simulink model "Lab40DEGREE"  (R2020a)
settings: Solver=VariableStepAuto  StartTime=0.0  StopTime=0.1  RelTol=1e-3
libraries: powerlib x17
settings Model: Creator=Ahmad Raza  LastModifiedBy=Dell

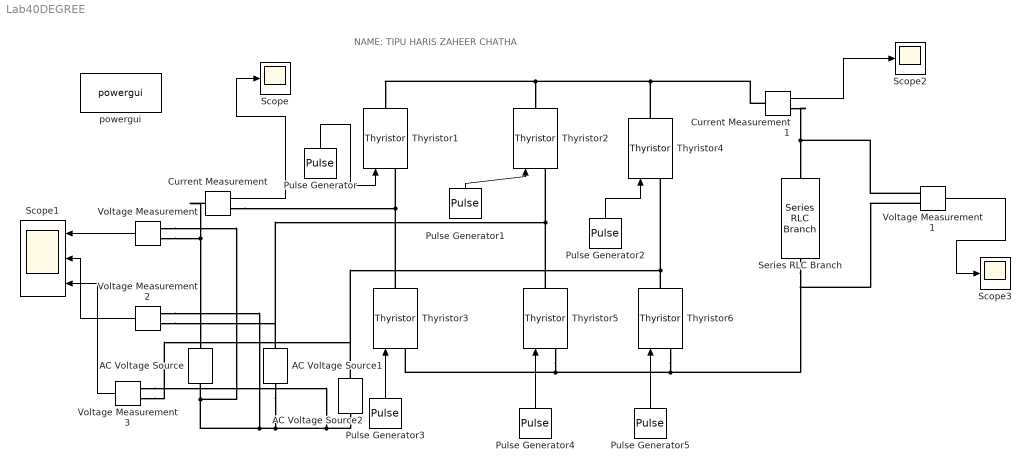
== system Lab40DEGREE ==
  note: NAME: TIPU HARIS ZAHEER CHATHA
  AC Voltage Source : powerlib/Electrical Sources/AC Voltage Source  Amplitude=100  Phase=0  Frequency=50  SampleTime=0  Measurements=None  BusType=swing  Pref=10e3  Qref=0  Qmin=-inf  Qmax=+inf
  AC Voltage Source1 : powerlib/Electrical Sources/AC Voltage Source  Amplitude=100  Phase=120  Frequency=50  SampleTime=0  Measurements=None  BusType=swing  Pref=10e3  Qref=0  Qmin=-inf  Qmax=+inf
  AC Voltage Source2 : powerlib/Electrical Sources/AC Voltage Source  Amplitude=100  Phase=240  Frequency=50  SampleTime=0  Measurements=None  BusType=swing  Pref=10e3  Qref=0  Qmin=-inf  Qmax=+inf
  Current Measurement : powerlib/Measurements/Current Measurement  PhasorSimulation=off  OutputType=Complex  PSBequivalent=0
  Current Measurement1 : powerlib/Measurements/Current Measurement  PhasorSimulation=off  OutputType=Complex  PSBequivalent=0
  Pulse Generator : DiscretePulseGenerator  PulseType=Time based  Amplitude=10  Period=0.02  PulseWidth=33.33  PhaseDelay=0/(360*50)
  Pulse Generator1 : DiscretePulseGenerator  PulseType=Time based  Amplitude=10  Period=0.02  PulseWidth=33.33  PhaseDelay=120/(360*50)
  Pulse Generator2 : DiscretePulseGenerator  PulseType=Time based  Amplitude=10  Period=0.02  PulseWidth=33.33  PhaseDelay=240/(360*50)
  Pulse Generator3 : DiscretePulseGenerator  PulseType=Time based  Amplitude=10  Period=0.02  PulseWidth=33.33  PhaseDelay=300/(360*50)
  Pulse Generator4 : DiscretePulseGenerator  PulseType=Time based  Amplitude=10  Period=0.02  PulseWidth=33.33  PhaseDelay=60/(360*50)
  Pulse Generator5 : DiscretePulseGenerator  PulseType=Time based  Amplitude=10  Period=0.02  PulseWidth=33.33  PhaseDelay=180/(360*50)
  Scope : Scope
  Scope1 : Scope  NumInputPorts=3
  Scope2 : Scope
  Scope3 : Scope
  Series RLC Branch : powerlib/Elements/Series RLC Branch  LConnTagsString=__new0  RConnTagsString=__new0  BranchType=R  Resistance=1  Inductance=1e-3  SetiL0=off  InitialCurrent=0  Capacitance=1e-6  Setx0=off  InitialVoltage=0  Measurements=None
  Thyristor{1..6} (6 alike) : powerlib/Power Electronics/Thyristor  Ron=0.001  Lon=0  Vf=0.8  IC=0  Rs=500  Cs=250e-9  Measurements=off
  Voltage Measurement{,1..3} (4 alike) : powerlib/Measurements/Voltage Measurement  PhasorSimulation=off  OutputType=Complex  PSBequivalent=0
  powergui : powerlib/powergui  Priority=1  SimulationMode=Continuous  SampleTime=50e-6  frequency=60  Iterations=50  frequencyindice=50  Pbase=100e6  ErrMax=1e-4  UnitsV=kV  UnitsW=MW  buscounter=0  FunctionMessages=off  echomessages=off  EnableUseOfTLC=off  CurrentSourceSwitches=off  DisableSnubberDevices=off  DisableRonSwitches=off  DisableVfSwitches=off  DisplayEquations=off  AutomaticDiscreteSolvers=off  SolverType=Tustin/Backward Euler (TBE)  Interpol=off  ExternalGateDelay=off  methode=off  Ts=100  x0status=blocks  SPID=on  SwTol=0  HookPort=off  NonlinearTolerance=1e-4  nMaxIteration=100  ContinueOnMaxIteration=off  RestoreLinks=warning  ResistiveCurrentMeasurement=off  Frange=[0:2:500]  Ylog=off  Xlog=on  ShowGrid=off  save=off  variable=ZData  structure=0  ZoomFFT=off  StartTime=0.0  cycles=1  DisplayStyle=1  fundamental=60  FreqAxis=off  MaxFrequency=1000  frequencyindicesteady=1  RmsSteady=1  display=off
  wires:
  Current Measurement/1 -> Scope/1
  Pulse Generator/1 -> Thyristor1/1
  Pulse Generator1/1 -> Thyristor2/1
  Pulse Generator2/1 -> Thyristor4/1
  Pulse Generator3/1 -> Thyristor3/1
  Pulse Generator4/1 -> Thyristor5/1
  Pulse Generator5/1 -> Thyristor6/1
  Current Measurement1/1 -> Scope2/1
  Voltage Measurement1/1 -> Scope3/1
  Voltage Measurement/1 -> Scope1/1
  Voltage Measurement2/1 -> Scope1/2
  Voltage Measurement3/1 -> Scope1/3
  connections:
  Thyristor3/RConn1 -- Current Measurement/RConn1 -- Thyristor1/LConn1
  Thyristor5/RConn1 -- Voltage Measurement2/LConn1 -- AC Voltage Source1/RConn1 -- Thyristor2/LConn1
  Thyristor6/RConn1 -- Voltage Measurement3/LConn1 -- AC Voltage Source2/RConn1 -- Thyristor4/LConn1
  AC Voltage Source2/LConn1 -- Voltage Measurement3/LConn2 -- AC Voltage Source1/LConn1 -- Voltage Measurement2/LConn2 -- Voltage Measurement/LConn2 -- AC Voltage Source/LConn1
  Current Measurement/LConn1 -- AC Voltage Source/RConn1 -- Voltage Measurement/LConn1
  Current Measurement1/LConn1 -- Thyristor4/RConn1 -- Thyristor2/RConn1 -- Thyristor1/RConn1
  Thyristor6/LConn1 -- Series RLC Branch/RConn1 -- Voltage Measurement1/LConn2 -- Thyristor5/LConn1 -- Thyristor3/LConn1
  Current Measurement1/RConn1 -- Voltage Measurement1/LConn1 -- Series RLC Branch/LConn1
